simulink model "Scope_can_read"  (R2020a)
settings: Solver=FixedStepAuto  StartTime=0.0  StopTime=inf  RelTol=1e-3  EnableMultiTasking=on
libraries: arduinolib x7, etargetslib x3
settings Model: SILPILModeSetting=veronly  ExtModeTrigDuration=2  Creator=imkis  LastModifiedBy=imkis
settings OptimizationCC: EnhancedBackFolding=on  PassReuseOutputArgsAs=Individual arguments  ZeroExternalMemoryAtStartup=off  ZeroInternalMemoryAtStartup=off  MaxStackSize=64  OptimizeBlockOrder=speed  DifferentSizesBufferReuse=on  OptimizationCustomize=off  EfficientTunableParamExpr=on
settings DebuggingCC: ParameterTunabilityLossMsg=error
settings HardwareCC: ProdBitPerInt=16  ProdBitPerPointer=16  ProdBitPerSizeT=16  ProdBitPerPtrDiffT=16  ProdLargestAtomicFloat=None  ProdWordSize=8  ProdHWDeviceType=Atmel->AVR
settings SFSimCC: MATLABDynamicMemAlloc=off
settings RTWCC: SystemTargetFile=ert.tlc  HardwareBoard=Arduino Mega 2560  TLCOptions=-aInlineSetEventsForThisBaseRateFcn=TLC_FALSE -aSuppressMultiTaskScheduler=TLC_FALSE -aRateBasedStepFcn=1  TemplateMakefile=ert_default_tmf  Toolchain=Arduino AVR  BuildConfiguration=Faster Runs
settings CodeAppCC: ForceParamTrailComments=on  IgnoreCustomStorageClasses=off  OperatorAnnotations=on  SimulinkDataObjDesc=on  SFDataObjDesc=on  InsertBlockDesc=on
settings ERTTargetCC: SupportContinuousTime=on  SupportVariableSizeSignals=on  ExtModeStaticAllocSize=2048

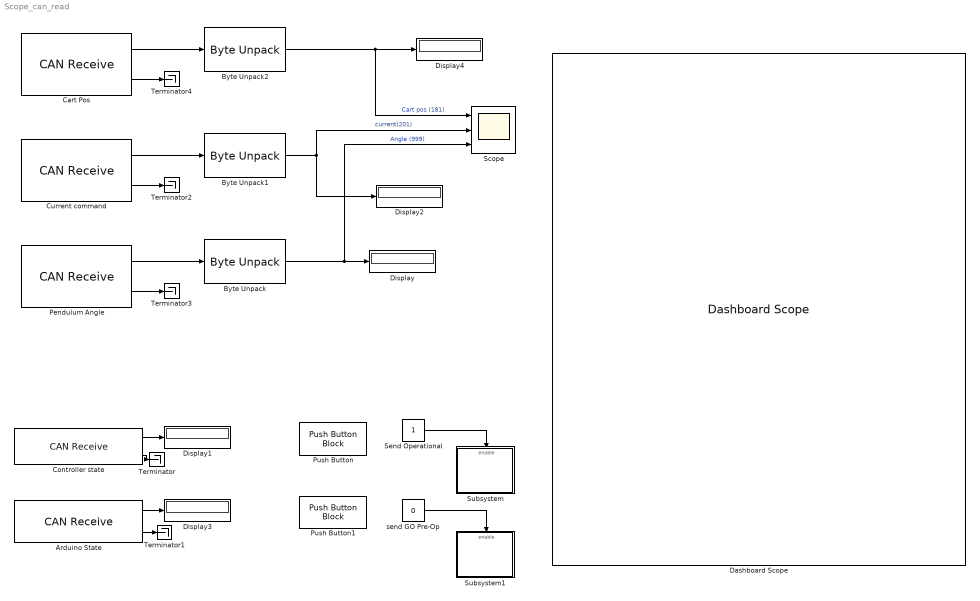
== system Scope_can_read ==
  Arduino State : arduinolib/CAN Receive  outputDataType=Raw data  identifierType=Standard (11-bit identifier)  messageId=hex2dec('702')  msgLength=1  SampleTime=1  outputError=off  outputRemote=off
      settings: SourceProductBaseCode=ARDUINO
  Byte Unpack : etargetslib/Byte Unpack  dimensions={[1]}  datatypes={'int32'}  byteAlign=4
  Byte Unpack1 : etargetslib/Byte Unpack  dimensions={[1]}  datatypes={'int16'}  byteAlign=2
  Byte Unpack2 : etargetslib/Byte Unpack  dimensions={[1]}  datatypes={'int32'}  byteAlign=4
  Cart Pos : arduinolib/CAN Receive  outputDataType=Raw data  identifierType=Standard (11-bit identifier)  messageId=hex2dec('181')  msgLength=4  SampleTime=0.001  outputError=off  outputRemote=off
      settings: SourceProductBaseCode=ARDUINO
  Controller state : arduinolib/CAN Receive  outputDataType=Raw data  identifierType=Standard (11-bit identifier)  messageId=hex2dec('701')  msgLength=1  SampleTime=1  outputError=off  outputRemote=off
      settings: SourceProductBaseCode=ARDUINO
  Current command : arduinolib/CAN Receive  outputDataType=Raw data  identifierType=Standard (11-bit identifier)  messageId=hex2dec('201')  msgLength=2  SampleTime=0.001  outputError=off  outputRemote=off
      settings: SourceProductBaseCode=ARDUINO
  Dashboard Scope : DashboardScope  Ymin=-1000  Ymax=1000
  Display{,1..4} (5 alike) : Display
  Pendulum Angle : arduinolib/CAN Receive  outputDataType=Raw data  identifierType=Standard (11-bit identifier)  messageId=999  msgLength=4  SampleTime=0.001  outputError=off  outputRemote=off
      settings: SourceProductBaseCode=ARDUINO
  Push Button : PushButtonBlock  ButtonText=Go Operational
  Push Button1 : PushButtonBlock  ButtonText=GO Pre-Operational
  Scope : Scope  NumInputPorts=3
  Send Operational : Constant
  Subsystem : Subsystem
  Subsystem1 : Subsystem
  Terminator{,1..4} (5 alike) : Terminator
  send GO Pre-Op : Constant  Value=0
  wires:
  Pendulum Angle/1 -> Byte Unpack/1
  Byte Unpack/1 -> Display/1, Scope/3  "Angle (999)"
  Arduino State/2 -> Terminator1/1
  send GO Pre-Op/1 -> Subsystem1/Enable
  Controller state/1 -> Display1/1
  Send Operational/1 -> Subsystem/Enable
  Arduino State/1 -> Display3/1
  Controller state/2 -> Terminator/1
  Pendulum Angle/2 -> Terminator3/1
  Current command/2 -> Terminator2/1
  Byte Unpack1/1 -> Display2/1, Scope/2  "current(201)"
  Current command/1 -> Byte Unpack1/1
  Cart Pos/2 -> Terminator4/1
  Byte Unpack2/1 -> Display4/1, Scope/1  "Cart pos (181)"
  Cart Pos/1 -> Byte Unpack2/1

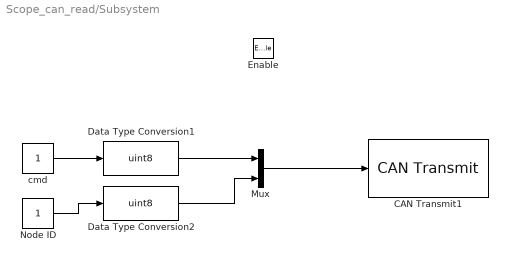
== system Scope_can_read/Subsystem ==
  Enable : EnablePort
  CAN Transmit1 : arduinolib/CAN Transmit  inputDataType=Raw data  BlockingMode_=off  BlockTimeout_=1  outputStatus=off  identifierType=Standard (11-bit identifier)  messageId=0  msgLength=2  remoteFrame=off
      settings: SourceProductBaseCode=ARDUINO
  Data Type Conversion1 : DataTypeConversion  OutDataTypeStr=uint8
  Data Type Conversion2 : DataTypeConversion  OutDataTypeStr=uint8
  Mux : Mux  Inputs=2
  Node ID : Constant  SampleTime=2
  cmd : Constant  SampleTime=2
  wires:
  Data Type Conversion2/1 -> Mux/2
  Data Type Conversion1/1 -> Mux/1
  Mux/1 -> CAN Transmit1/1
  Node ID/1 -> Data Type Conversion2/1
  cmd/1 -> Data Type Conversion1/1

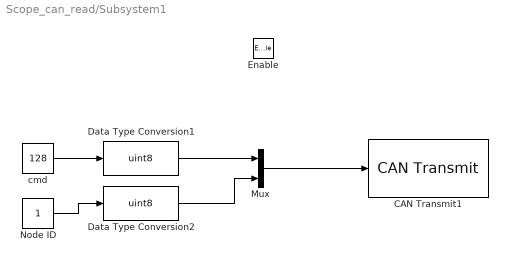
== system Scope_can_read/Subsystem1 ==
  Enable : EnablePort
  CAN Transmit1 : arduinolib/CAN Transmit  inputDataType=Raw data  BlockingMode_=off  BlockTimeout_=1  outputStatus=off  identifierType=Standard (11-bit identifier)  messageId=0  msgLength=2  remoteFrame=off
      settings: SourceProductBaseCode=ARDUINO
  Data Type Conversion1 : DataTypeConversion  OutDataTypeStr=uint8
  Data Type Conversion2 : DataTypeConversion  OutDataTypeStr=uint8
  Mux : Mux  Inputs=2
  Node ID : Constant  SampleTime=1
  cmd : Constant  Value=128  SampleTime=1
  wires:
  Data Type Conversion2/1 -> Mux/2
  Data Type Conversion1/1 -> Mux/1
  Mux/1 -> CAN Transmit1/1
  Node ID/1 -> Data Type Conversion2/1
  cmd/1 -> Data Type Conversion1/1
